simulink model "Modelo_practica4"  (R2021a)
settings: Solver=VariableStepAuto  StartTime=0.0  StopTime=5  MaxStep=1e-5  RelTol=1e-3
values from neighbouring files (symbols this model uses):
  A = [0  1; 0  -125.59]    [modelo_ideal_Practica6.mat]    (also in modelo_practica4_workspace.mat; modelo_real_practica5_workspace.mat)
  B = [0 132500]    [modelo_ideal_Practica6.mat]    (also in modelo_practica4_workspace.mat; modelo_real_practica5_workspace.mat)
  C = [1 0]    [modelo_ideal_Practica6.mat]    (also in modelo_practica4_workspace.mat; modelo_real_practica5_workspace.mat)
  K = [-3.78656830443e-05 4.70346663172e-05]    [modelo_ideal_Practica6.mat]    (also in modelo_practica4_workspace.mat = [0.0297600907547 -0.00189569811321]; modelo_real_practica5_workspace.mat)
  k_e = 132500    [modelo_ideal_Practica6.mat]    (also in modelo_ideal_practica3_workspace.mat; modelo_practica4_workspace.mat; modelo_real_practica5_workspace.mat)
  L = [-1.20402629539 1.69403138607]    [modelo_ideal_Practica6.mat]    (also in modelo_practica4_workspace.mat = [-251.18 35488.908225]; modelo_real_practica5_workspace.mat)
  p = 125.59    [modelo_ideal_Practica6.mat]    (also in modelo_ideal_practica3_workspace.mat; modelo_practica4_workspace.mat; modelo_real_practica5_workspace.mat)
settings Model: Creator=Marcial  LastModifiedBy=Marcial

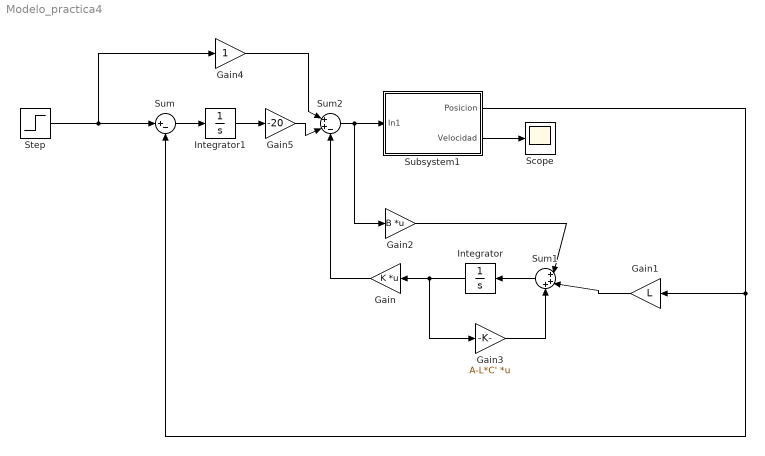
== system Modelo_practica4 ==
  Gain : Gain  Gain=K  Multiplication=Matrix(K*u)
  Gain1 : Gain  Gain=L
  Gain2 : Gain  Gain=B  Multiplication=Matrix(K*u)
  Gain3 : Gain  Gain=A-L*C'  Multiplication=Matrix(K*u)
  Gain4 : Gain
  Gain5 : Gain  Gain=-20
  Integrator : Integrator
  Integrator1 : Integrator
  Scope : Scope
  Step : Step  Time=0  SampleTime=0
  Subsystem1 : Subsystem
  Sum : Sum  Inputs=|+-
  Sum1 : Sum  Inputs=|+++
  Sum2 : Sum  Inputs=|++-
  wires:
  Subsystem1/2(Velocidad) -> Scope/1
  Step/1 -> Gain4/1, Sum/1
  Gain2/1 -> Sum1/1
  Gain1/1 -> Sum1/2
  Sum1/1 -> Integrator/1
  Integrator/1 -> Gain/1, Gain3/1
  Gain3/1 -> Sum1/3
  Integrator1/1 -> Gain5/1
  Sum/1 -> Integrator1/1
  Sum2/1 -> Gain2/1, Subsystem1/1(In1)
  Gain5/1 -> Sum2/2
  Gain4/1 -> Sum2/1
  Gain/1 -> Sum2/3
  Subsystem1/1(Posicion) -> Sum/2, Gain1/1

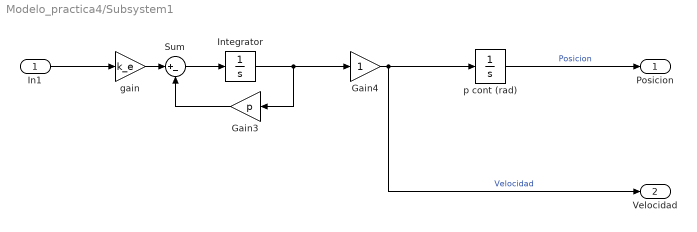
== system Modelo_practica4/Subsystem1 ==
  In1 : Inport
  Gain3 : Gain  Gain=p
  Gain4 : Gain
  Integrator : Integrator
  Sum : Sum  Inputs=|+-
  gain : Gain  Gain=k_e
  p cont (rad) : Integrator
  Posicion : Outport
  Velocidad : Outport  Port=2
  wires:
  Integrator/1 -> Gain3/1, Gain4/1
  Gain3/1 -> Sum/2
  gain/1 -> Sum/1
  Gain4/1 -> Velocidad/1, p cont (rad)/1  "Velocidad"
  Sum/1 -> Integrator/1
  p cont (rad)/1 -> Posicion/1  "Posicion"
  In1/1 -> gain/1
